simulink model "flc_picomotor"  (R2014a)
settings: Solver=ode45  StartTime=0.0  StopTime=100  RelTol=1e-3
libraries: fuzblock x1
settings Model: Creator=KRISH  LastModifiedBy=KRISH

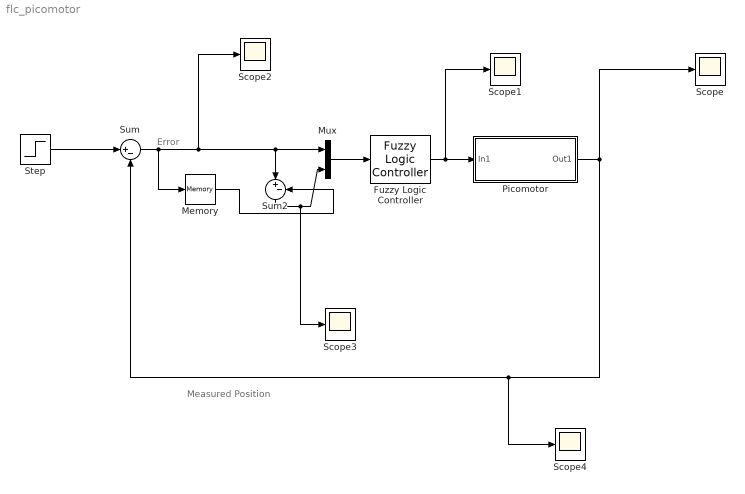
== system flc_picomotor ==
  note: Error
  note: Measured Position
  Fuzzy Logic Controller : fuzblock/Fuzzy Logic  Controller  fis='flc_pid2.fis'
  Memory : Memory
  Mux : Mux  Inputs=2
  "Picomotor " : Subsystem
  Scope{,1..4} (5 alike) : Scope
      Scope settings: TimeRange=0.001966153848734442  YMin=0.4783320787422278  YMax=0.4895433515597992  SaveName=ScopeData2
      Scope1 settings: SaveName=ScopeData3
      Scope2 settings: SaveName=ScopeData4
      Scope3 settings: SaveName=ScopeData5
      Scope4 settings: TimeRange=0.001966153848734442  YMin=0.4783320787422278  YMax=0.4895433515597992
  Step : Step  Before=-6  After=6  SampleTime=2  VectorParams1D=off  ZeroCross=off
  Sum : Sum  Inputs=|+-
  Sum2 : Sum  Inputs=|+-
  wires:
  Fuzzy Logic Controller/1 -> Scope1/1, "Picomotor "/1(In1)
  Sum/1 -> Memory/1, Scope2/1, Sum2/1, Mux/1
  Memory/1 -> Sum2/2
  Mux/1 -> Fuzzy Logic Controller/1
  Sum2/1 -> Scope3/1, Mux/2
  "Picomotor "/1(Out1) -> Scope4/1, Sum/2, Scope/1
  Step/1 -> Sum/1

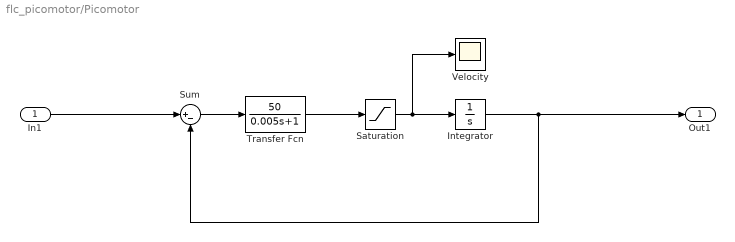
== system flc_picomotor/Picomotor  ==
  In1 : Inport  OutMin=-6  OutMax=6
  Integrator : Integrator
  Saturation : Saturate
  Sum : Sum  Inputs=|+-
  Transfer Fcn : TransferFcn  Numerator=[50]  Denominator=[0.005 1]
  Velocity : Scope
      settings: TimeRange=10
  Out1 : Outport
  wires:
  Transfer Fcn/1 -> Saturation/1
  Saturation/1 -> Velocity/1, Integrator/1
  Integrator/1 -> Sum/2, Out1/1
  Sum/1 -> Transfer Fcn/1
  In1/1 -> Sum/1
